simulink model "model"  (R2022a)
settings: Solver=ode4  StartTime=0.0  StopTime=20.0  FixedStep=1e-3  RelTol=1e-3
values from neighbouring files (symbols this model uses):
  d = 44.51e-3    (= 0.04451)    [simulateModel.m]
  I = Ic + mc*d^2 + 2*mw*L^2 + 2*Im    (= 0.2786255713)    [simulateModel.m]
  Iw = 40e-3    (= 0.04)    [simulateModel.m]
  Kb = 23e-3    (= 0.023)    [simulateModel.m]
  Kt = 29e-3    (= 0.029)    [simulateModel.m]
  L = 0.1655    [simulateModel.m]
  La = 0.66e-3    (= 0.00066)    [simulateModel.m]
  m = mc + 2*mw    (= 16)    [simulateModel.m]
  mc = 13    [simulateModel.m]
  N = 38.3    [simulateModel.m]
  R = D/2    (= 0.0975)    [simulateModel.m]
  Ra = 710e-3    (= 0.71)    [simulateModel.m]
undefined symbols (not defined in the file or in its folder): sigbuilder_block
libraries: simulink x5
settings Model: Creator=mateu  LastModifiedBy=mateu

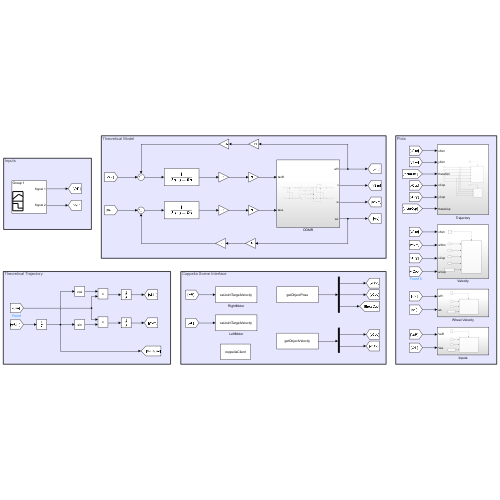
[thumbnail: Simulink's stored preview of the top-level diagram]
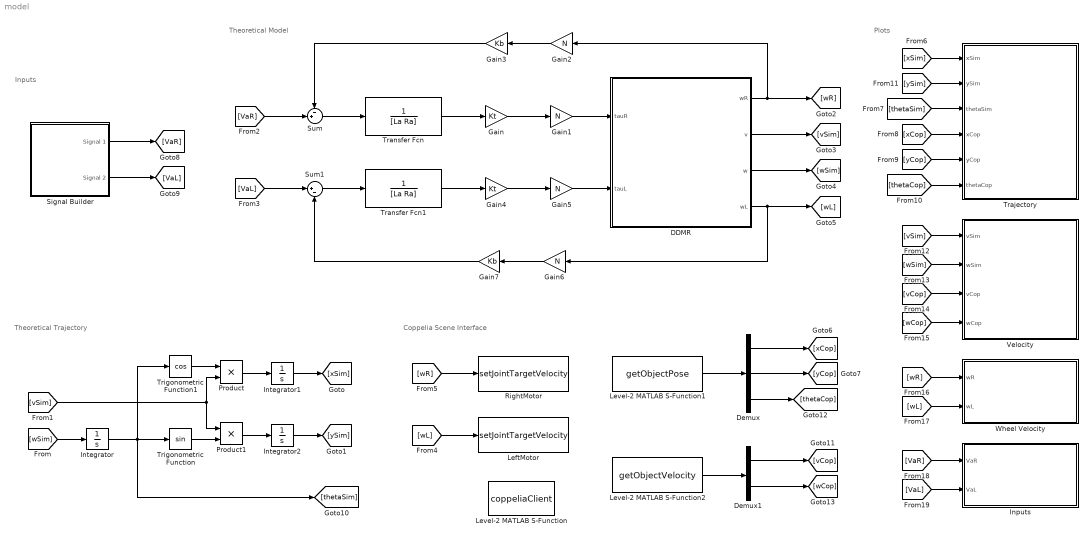
== system model ==
  note: Plots
  note: Coppelia Scene Interface
  note: Theoretical Trajectory
  note: Theoretical Model
  note: Inputs
  DDMR : Subsystem
  Demux : Demux  Outputs=3
  Demux1 : Demux  Outputs=2
  Gain : Gain  Gain=Kt
  Gain{1..2,5..6} (4 alike) : Gain  Gain=N
  Gain3 : Gain  Gain=Kb
  Gain4 : Gain  Gain=Kt
  Gain7 : Gain  Gain=Kb
  Inputs : Subsystem
  Integrator : Integrator
  Integrator1 : Integrator
  Integrator2 : Integrator
  LeftMotor : M-S-Function  FunctionName=setJointTargetVelocity  Parameters='/PioneerP3DX/leftMotor'
  Level-2 MATLAB S-Function : M-S-Function  FunctionName=coppeliaClient  Parameters=true
  Level-2 MATLAB S-Function1 : M-S-Function  FunctionName=getObjectPose  Parameters='/PioneerP3DX'
  Level-2 MATLAB S-Function2 : M-S-Function  FunctionName=getObjectVelocity  Parameters='/PioneerP3DX'
  Product : Product
  Product1 : Product
  RightMotor : M-S-Function  FunctionName=setJointTargetVelocity  Parameters='/PioneerP3DX/rightMotor'
  Signal Builder : Subsystem  Tag=STV Subsys  LoadFcn=sigbuilder_block('load');  StartFcn=sigbuilder_block('start');  StopFcn=sigbuilder_block('stop');  ClipboardFcn=sigbuilder_block('clipboard');  mask(Sigbuilder block){tuvar=[0:10]}
      mask help: Simulink:masks:SigbuilderBlock_MD
      mask init:
      | if ~strcmp(get_param(bdroot(gcbh),'SimulationStatus'),'stopped') tuvar = sigbuilder_block('maskInit'); end
      settings: CopyFcn=sigbuilder_block('copy');  DeleteFcn=sigbuilder_block('delete');  ModelCloseFcn=sigbuilder_block('modelClose');  PreSaveFcn=sigbuilder_block('preSave');  PauseFcn=sigbuilder_block('pause');  ContinueFcn=sigbuilder_block('continue');  NameChangeFcn=sigbuilder_block('namechange');  OpenFcn=sigbuilder_block('open',[437.6 199.2 550.4 400 ]);  CloseFcn=sigbuilder_block('close');
      mask Display: plot(0, 0, 100, 100,[2, 2, 32, 32, 2], [68, 8, 8, 68, 68],[32, 2], [38, 38], [32, 19, 2],[53, 60, 44], [32, 17, 17, 2],[16, 16, 31, 31]);txt = getActiveGroup(gcbh);text(2, 100, txt,'verticalAlignment', 'top');
  Sum : Sum  Inputs=-+|
  Sum1 : Sum  Inputs=|+-
  Trajectory : Subsystem
  Transfer Fcn : TransferFcn  Denominator=[La Ra]
  Transfer Fcn1 : TransferFcn  Denominator=[La Ra]
  Trigonometric Function : Trigonometry
  Trigonometric Function1 : Trigonometry  Operator=cos
  Velocity : Subsystem
  Wheel Velocity : Subsystem
  wires:
  Transfer Fcn/1 -> Gain/1
  Gain/1 -> Gain1/1
  Gain1/1 -> DDMR/1(tauR)
  Sum/1 -> Transfer Fcn/1
  Gain2/1 -> Gain3/1
  Gain3/1 -> Sum/1
  DDMR/1(wR) -> [wR], Gain2/1
  Transfer Fcn1/1 -> Gain4/1
  Gain4/1 -> Gain5/1
  Gain5/1 -> DDMR/2(tauL)
  Sum1/1 -> Transfer Fcn1/1
  Gain6/1 -> Gain7/1
  DDMR/4(wL) -> [wL], Gain6/1
  Gain7/1 -> Sum1/2
  Product/1 -> Integrator1/1
  Product1/1 -> Integrator2/1
  Trigonometric Function1/1 -> Product/1
  [vSim] -> Product1/1, Product/2
  Integrator/1 -> [thetaSim], Trigonometric Function1/1, Trigonometric Function/1
  Trigonometric Function/1 -> Product1/2
  [wSim] -> Integrator/1
  Integrator1/1 -> [xSim]
  Integrator2/1 -> [ySim]
  DDMR/2(v) -> [vSim]
  DDMR/3(w) -> [wSim]
  [VaR] -> Sum/2
  [VaL] -> Sum1/1
  [wR] -> RightMotor/1
  [wL] -> LeftMotor/1
  Level-2 MATLAB S-Function1/1 -> Demux/1
  Demux/3 -> [thetaCop]
  Demux/1 -> [xCop]
  Demux/2 -> [yCop]
  Signal Builder/1(Signal 1) -> [VaR]
  Level-2 MATLAB S-Function2/1 -> Demux1/1
  Demux1/2 -> [wCop]
  Demux1/1 -> [vCop]
  [xSim] -> Trajectory/1(xSim)
  [ySim] -> Trajectory/2(ySim)
  [thetaSim] -> Trajectory/3(thetaSim)
  [xCop] -> Trajectory/4(xCop)
  [yCop] -> Trajectory/5(yCop)
  [thetaCop] -> Trajectory/6(thetaCop)
  [vSim] -> Velocity/1(vSim)
  [wSim] -> Velocity/2(wSim)
  [vCop] -> Velocity/3(vCop)
  [wCop] -> Velocity/4(wCop)
  Signal Builder/2(Signal 2) -> [VaL]
  [wR] -> Wheel Velocity/1(wR)
  [wL] -> Wheel Velocity/2(wL)
  [VaR] -> Inputs/1(VaR)
  [VaL] -> Inputs/2(VaL)

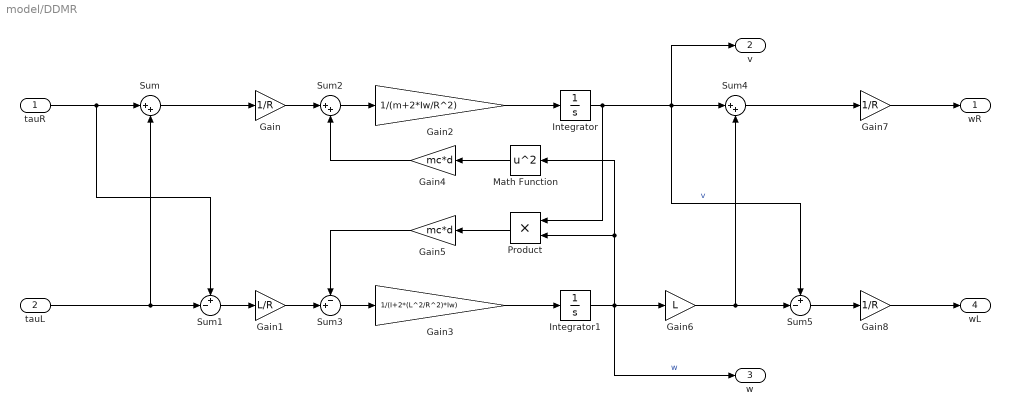
== system model/DDMR ==
  tauR : Inport
  tauL : Inport  Port=2
  Gain : Gain  Gain=1/R
  Gain1 : Gain  Gain=L/R
  Gain2 : Gain  Gain=1/(m+2*Iw/R^2)
  Gain3 : Gain  Gain=1/(I+2*(L^2/R^2)*Iw)
  Gain4 : Gain  Gain=mc*d
  Gain5 : Gain  Gain=mc*d
  Gain6 : Gain  Gain=L
  Gain7 : Gain  Gain=1/R
  Gain8 : Gain  Gain=1/R
  Integrator : Integrator
  Integrator1 : Integrator
  Math Function : Math  Operator=square
  Product : Product
  Sum : Sum  Inputs=|++
  Sum1 : Sum  Inputs=+-|
  Sum2 : Sum  Inputs=|++
  Sum3 : Sum  Inputs=-+|
  Sum4 : Sum  Inputs=|++
  Sum5 : Sum  Inputs=+-|
  wR : Outport
  v : Outport  Port=2
  w : Outport  Port=3
  wL : Outport  Port=4
  wires:
  Integrator1/1 -> w/1, Gain6/1, Product/2, Math Function/1  "w"
  tauL/1 -> Sum1/2, Sum/2
  Gain4/1 -> Sum2/2
  Gain6/1 -> Sum5/2, Sum4/2
  Integrator/1 -> v/1, Sum5/1, Sum4/1, Product/1  "v"
  Sum2/1 -> Gain2/1
  Gain7/1 -> wR/1
  Gain/1 -> Sum2/1
  Gain5/1 -> Sum3/1
  Sum1/1 -> Gain1/1
  Sum/1 -> Gain/1
  Math Function/1 -> Gain4/1
  Gain3/1 -> Integrator1/1
  Sum4/1 -> Gain7/1
  tauR/1 -> Sum/1, Sum1/1
  Product/1 -> Gain5/1
  Gain2/1 -> Integrator/1
  Sum5/1 -> Gain8/1
  Sum3/1 -> Gain3/1
  Gain1/1 -> Sum3/2
  Gain8/1 -> wL/1

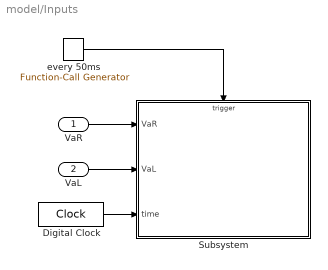
== system model/Inputs ==
  VaR : Inport
  VaL : Inport  Port=2
  Digital Clock : DigitalClock  SampleTime=50e-3
  Subsystem : Subsystem
  every 50ms : simulink/Ports & Subsystems/Function-Call Generator  sample_time=50e-3  numberOfIterations=1  DisallowWideOutput=off
  wires:
  VaL/1 -> Subsystem/2(VaL)
  every 50ms/1 -> Subsystem/Trigger
  VaR/1 -> Subsystem/1(VaR)
  Digital Clock/1 -> Subsystem/3(time)

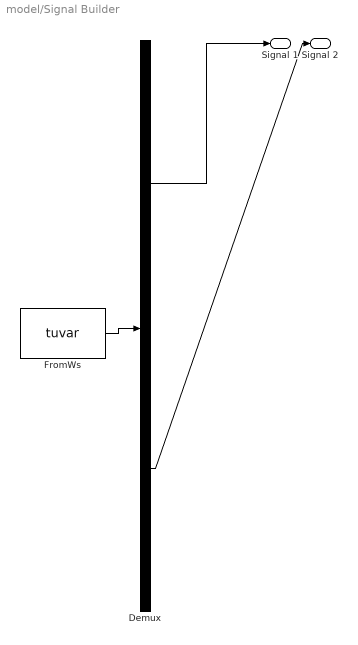
== system model/Signal Builder ==
  Demux : Demux  Tag=STV Demux  Outputs=2
      settings: DisplayOption=none
  FromWs : FromWorkspace  Tag=STV FromWs  VariableName=tuvar  OutputAfterFinalValue=Holding final value
      SigBuilderData=|
      | common.afterFinalStr = 'Hold final value'
      | common.sampleTime = '0'
      | dataSet.timeRange = [0 20]
      | dataSet.name = 'Group 1'
      | sbobj.Groups.Name = 'Group 1'
      | sbobj.Groups.Signals(1).Name = 'Signal 1'
      | sbobj.Groups.Signals(1).XData = [0 10 20]
      | sbobj.Groups.Signals(1).YData = [0 12 6]
      | sbobj.Groups.Signals(2).Name = 'Signal 2'
      | sbobj.Groups.Signals(2).XData = [0 10 20]
      | sbobj.Groups.Signals(2).YData = [0 10 10]
      | sbobj.Groups.TimeRange = [0 20]
  Signal 1 : Outport  Tag=STV Outport
  Signal 2 : Outport  Tag=STV Outport  Port=2
  wires:
  Demux/1 -> Signal 1/1
  FromWs/1 -> Demux/1
  Demux/2 -> Signal 2/1

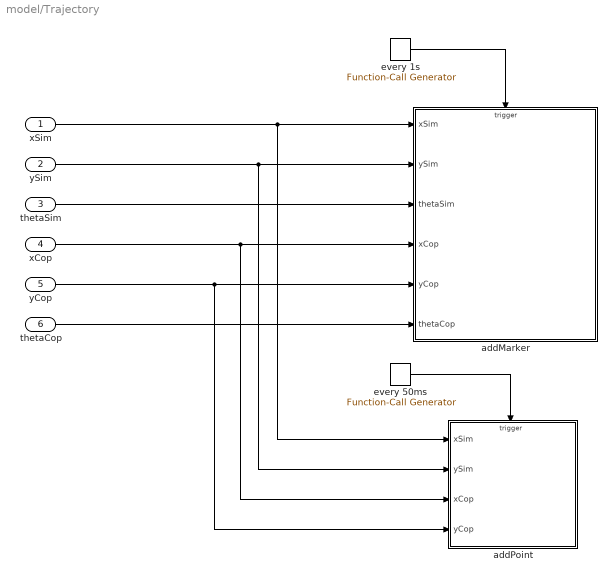
== system model/Trajectory ==
  xSim : Inport
  ySim : Inport  Port=2
  thetaSim : Inport  Port=3
  xCop : Inport  Port=4
  yCop : Inport  Port=5
  thetaCop : Inport  Port=6
  addMarker : Subsystem
  addPoint : Subsystem
  every 1s : simulink/Ports & Subsystems/Function-Call Generator  sample_time=1  numberOfIterations=1  DisallowWideOutput=off
  "every 50ms " : simulink/Ports & Subsystems/Function-Call Generator  sample_time=50e-3  numberOfIterations=1  DisallowWideOutput=off
  wires:
  xSim/1 -> addMarker/1(xSim), addPoint/1(xSim)
  ySim/1 -> addMarker/2(ySim), addPoint/2(ySim)
  thetaSim/1 -> addMarker/3(thetaSim)
  xCop/1 -> addMarker/4(xCop), addPoint/3(xCop)
  yCop/1 -> addPoint/4(yCop), addMarker/5(yCop)
  thetaCop/1 -> addMarker/6(thetaCop)
  every 1s/1 -> addMarker/Trigger
  "every 50ms "/1 -> addPoint/Trigger

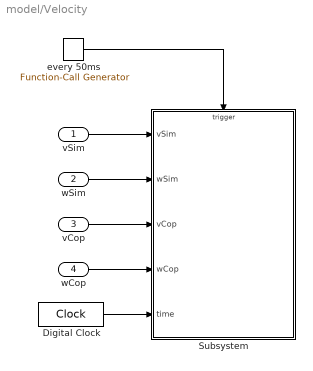
== system model/Velocity ==
  vSim : Inport
  wSim : Inport  Port=2
  vCop : Inport  Port=3
  wCop : Inport  Port=4
  Digital Clock : DigitalClock  SampleTime=50e-3
  Subsystem : Subsystem
  every 50ms : simulink/Ports & Subsystems/Function-Call Generator  sample_time=50e-3  numberOfIterations=1  DisallowWideOutput=off
  wires:
  every 50ms/1 -> Subsystem/Trigger
  vCop/1 -> Subsystem/3(vCop)
  wCop/1 -> Subsystem/4(wCop)
  wSim/1 -> Subsystem/2(wSim)
  vSim/1 -> Subsystem/1(vSim)
  Digital Clock/1 -> Subsystem/5(time)

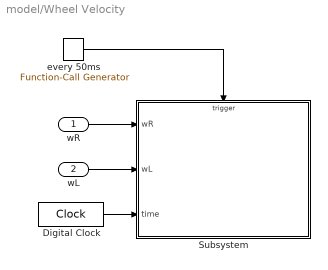
== system model/Wheel Velocity ==
  wR : Inport
  wL : Inport  Port=2
  Digital Clock : DigitalClock  SampleTime=50e-3
  Subsystem : Subsystem
  every 50ms : simulink/Ports & Subsystems/Function-Call Generator  sample_time=50e-3  numberOfIterations=1  DisallowWideOutput=off
  wires:
  wL/1 -> Subsystem/2(wL)
  every 50ms/1 -> Subsystem/Trigger
  wR/1 -> Subsystem/1(wR)
  Digital Clock/1 -> Subsystem/3(time)

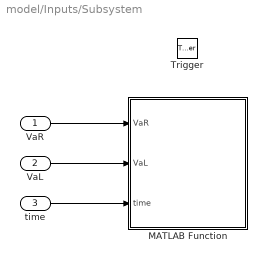
== system model/Inputs/Subsystem ==
  VaR : Inport
  VaL : Inport  Port=2
  time : Inport  Port=3
  Trigger : TriggerPort  TriggerType=function-call  VariantControl=(inherit)  PortDimensions=1
  MATLAB Function : MATLAB Function  TreatAsAtomicUnit=on
  wires:
  VaR/1 -> MATLAB Function/1(VaR)
  VaL/1 -> MATLAB Function/2(VaL)
  time/1 -> MATLAB Function/3(time)

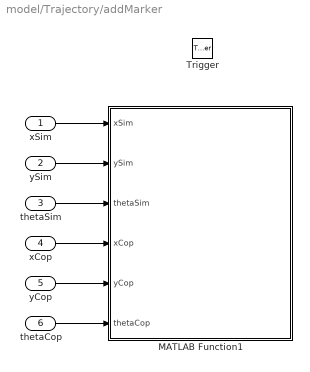
== system model/Trajectory/addMarker ==
  xSim : Inport
  ySim : Inport  Port=2
  thetaSim : Inport  Port=3
  xCop : Inport  Port=4
  yCop : Inport  Port=5
  thetaCop : Inport  Port=6
  Trigger : TriggerPort  TriggerType=function-call  VariantControl=(inherit)  PortDimensions=1
  MATLAB Function1 : MATLAB Function  TreatAsAtomicUnit=on
  wires:
  yCop/1 -> MATLAB Function1/5(yCop)
  xCop/1 -> MATLAB Function1/4(xCop)
  thetaSim/1 -> MATLAB Function1/3(thetaSim)
  thetaCop/1 -> MATLAB Function1/6(thetaCop)
  ySim/1 -> MATLAB Function1/2(ySim)
  xSim/1 -> MATLAB Function1/1(xSim)

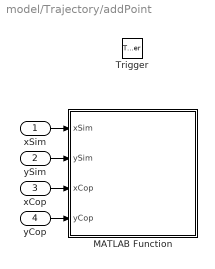
== system model/Trajectory/addPoint ==
  xSim : Inport
  ySim : Inport  Port=2
  xCop : Inport  Port=3
  yCop : Inport  Port=4
  Trigger : TriggerPort  TriggerType=function-call  VariantControl=(inherit)  PortDimensions=1
  MATLAB Function : MATLAB Function  TreatAsAtomicUnit=on
  wires:
  xSim/1 -> MATLAB Function/1(xSim)
  xCop/1 -> MATLAB Function/3(xCop)
  ySim/1 -> MATLAB Function/2(ySim)
  yCop/1 -> MATLAB Function/4(yCop)

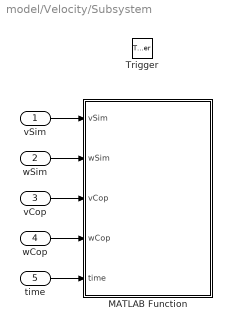
== system model/Velocity/Subsystem ==
  vSim : Inport
  wSim : Inport  Port=2
  vCop : Inport  Port=3
  wCop : Inport  Port=4
  time : Inport  Port=5
  Trigger : TriggerPort  TriggerType=function-call  VariantControl=(inherit)  PortDimensions=1
  MATLAB Function : MATLAB Function  TreatAsAtomicUnit=on
  wires:
  vSim/1 -> MATLAB Function/1(vSim)
  vCop/1 -> MATLAB Function/3(vCop)
  wSim/1 -> MATLAB Function/2(wSim)
  wCop/1 -> MATLAB Function/4(wCop)
  time/1 -> MATLAB Function/5(time)

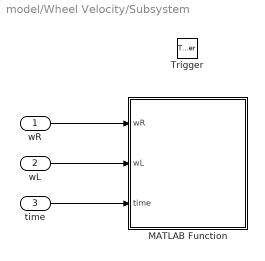
== system model/Wheel Velocity/Subsystem ==
  wR : Inport
  wL : Inport  Port=2
  time : Inport  Port=3
  Trigger : TriggerPort  TriggerType=function-call  VariantControl=(inherit)  PortDimensions=1
  MATLAB Function : MATLAB Function  TreatAsAtomicUnit=on
  wires:
  wR/1 -> MATLAB Function/1(wR)
  wL/1 -> MATLAB Function/2(wL)
  time/1 -> MATLAB Function/3(time)

== matlab function model/Trajectory/addMarker/MATLAB Function1 ==
  data: xSim input; ySim input; thetaSim input; xCop input; yCop input; thetaCop input
function addMarker(xSim,ySim,thetaSim,xCop,yCop,thetaCop)

coder.extrinsic('plotRobot');
plotRobot(xSim,ySim,thetaSim,xCop,yCop,thetaCop);

== matlab function model/Trajectory/addPoint/MATLAB Function ==
  data: xSim input; ySim input; xCop input; yCop input
function addPoint(xSim,ySim,xCop,yCop)

coder.extrinsic('plotPath');
plotPath(xSim,ySim,xCop,yCop);

== matlab function model/Velocity/Subsystem/MATLAB Function ==
  data: vSim input; wSim input; vCop input; wCop input; time input
function addVelPoint(vSim,wSim,vCop,wCop,time)

coder.extrinsic('plotVelocity');
plotVelocity(vSim,wSim,vCop,wCop,time);

== matlab function model/Wheel Velocity/Subsystem/MATLAB Function ==
  data: wR input; wL input; time input
function plotWheelVel(wR,wL,time)

coder.extrinsic('plotWheelVelocity');
plotWheelVelocity(wR,wL,time);

== matlab function model/Inputs/Subsystem/MATLAB Function ==
  data: VaR input; VaL input; time input
function plotInput(VaR,VaL,time)

coder.extrinsic('plotInputSignal');
plotInputSignal(VaR,VaL,time);
